simulink model "rotor_friction_coefficient_identification_model"  (R2024b)
settings: Solver=ode45  StartTime=0  StopTime=T(end)  MaxStep=0.01  RelTol=1e-3
values from neighbouring files (symbols this model uses):
  omega0 = 422.554608411    [currwork.mat]    (also in pendulum_friction_coefficient_identification.m = 0)
  uc_init = 0.001    [currwork.mat]    (also in pendulum_friction_coefficient_identification.m)
  uv_init = 0.001    [currwork.mat]    (also in pendulum_friction_coefficient_identification.m)
undefined symbols (not defined in the file or in its folder): J_rotor
settings Model: Creator=Student  LastModifiedBy=Paweł Wiktor
settings SolverCC: ZeroCrossControl=DisableAll  AlgebraicLoopSolver=TrustRegion
settings DataIOCC: ReturnWorkspaceOutputs=off
settings DebuggingCC: UnconnectedInputMsg=warning  UnconnectedOutputMsg=warning  UnconnectedLineMsg=warning  ArithmeticOperatorsInVariantConditions=warning
settings ModelReferenceCC: EnableRefExpFcnMdlSchedulingChecks=on
settings SFSimCC: CustomCodeUndefinedFunction=UseInterfaceOnly
settings RTWCC: GPUComputeCapability=3.5

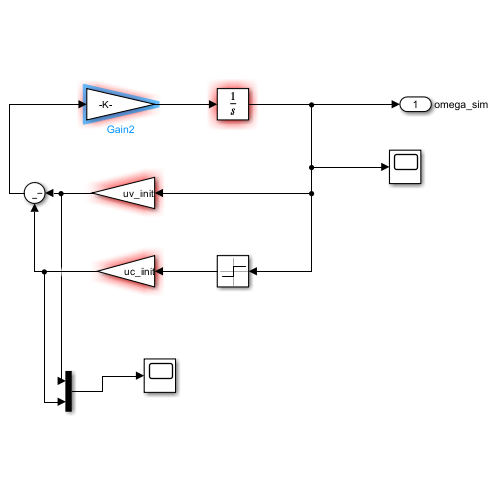
[thumbnail: Simulink's stored preview of the top-level diagram]
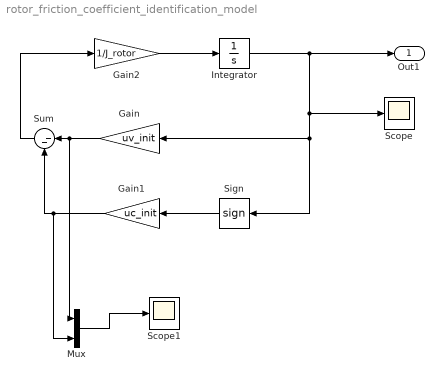
== system rotor_friction_coefficient_identification_model ==
  Gain : Gain  Gain=uv_init
  Gain1 : Gain  Gain=uc_init
  Gain2 : Gain  Gain=1/J_rotor
  Integrator : Integrator  InitialCondition=omega0
  Mux : Mux  Inputs=2
  Scope : Scope
  Scope1 : Scope
  Sign : Signum  ZeroCross=off
  Sum : Sum  Inputs=|--
  Out1 : Outport  SignalName=omega_sim  VectorParamsAs1DForOutWhenUnconnected=off
  wires:
  Gain/1 -> Mux/1, Sum/1
  Gain1/1 -> Mux/2, Sum/2
  Sign/1 -> Gain1/1
  Sum/1 -> Gain2/1
  Gain2/1 -> Integrator/1
  Integrator/1 -> Gain/1, Sign/1, Scope/1, Out1/1
  Mux/1 -> Scope1/1
